simulink model "Problem_5"  (R2020a)
settings: Solver=VariableStepAuto  StartTime=0.0  StopTime=30  RelTol=1e-3
model workspace (MAT data in the model file):
  C = Simulink.Parameter
  C.Value = 10
  C.DataType = 'auto'
  C.Dimensions = [1 1]
  R = Simulink.Parameter
  R.Value = 10
  R.DataType = 'auto'
  R.Dimensions = [1 1]
settings Model: Creator=hp  LastModifiedBy=hp

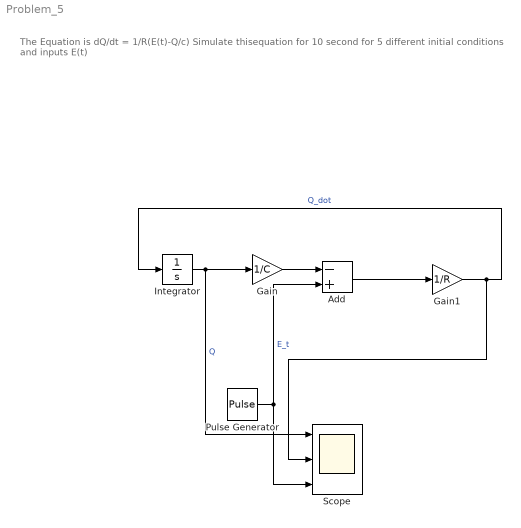
== system Problem_5 ==
  note: The Equation is
      | dQ/dt = 1/R(E(t)-Q/c)
      | Simulate thisequation for 10 second for 5 different initial conditions and inputs E(t)
  Add : Sum  Inputs=-+
  Gain : Gain  Gain=1/C
  Gain1 : Gain  Gain=1/R
  Integrator : Integrator
  Pulse Generator : DiscretePulseGenerator  PulseType=Time based  Period=10  PulseWidth=5
  Scope : Scope  NumInputPorts=3
  wires:
  Gain/1 -> Add/1
  Integrator/1 -> Scope/1, Gain/1  "Q"
  Add/1 -> Gain1/1
  Gain1/1 -> Integrator/1, Scope/2  "Q_dot"
  Pulse Generator/1 -> Scope/3, Add/2  "E_t"
